simulink model "untitled"  (R2020a)
settings: Solver=VariableStepAuto  StartTime=0.0  StopTime=10.0  RelTol=1e-3
values from neighbouring files (symbols this model uses):
  tmax = 32    [matlab.mat]
  tmin = -26    [matlab.mat]
libraries: mpclib x1
settings Model: Creator=lamarre  LastModifiedBy=lamarre

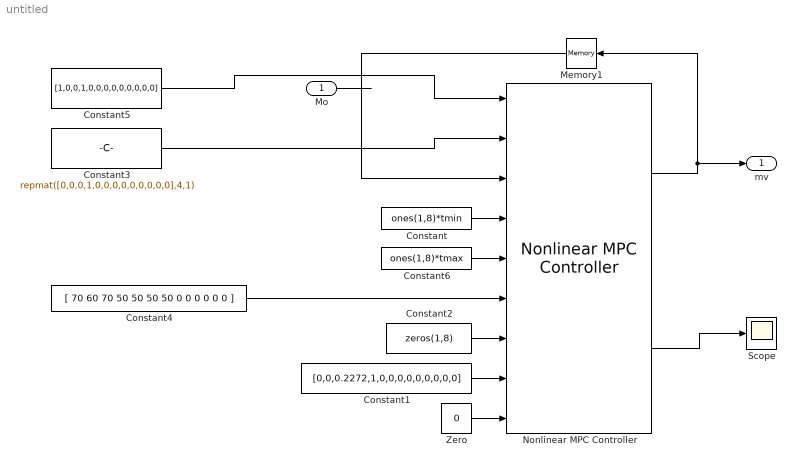
== system untitled ==
  Mo : Inport
  Constant : Constant  Value=ones(1,8)*tmin  VectorParams1D=off
  Constant1 : Constant  Value=[0,0,0.2272,1,0,0,0,0,0,0,0,0,0]  VectorParams1D=off
  Constant2 : Constant  Value=zeros(1,8)  VectorParams1D=off
  Constant3 : Constant  Value=repmat([0,0,0,1,0,0,0,0,0,0,0,0,0],4,1)  VectorParams1D=off
  Constant4 : Constant  Value=[ 70 60 70 50 50 50 50 0 0 0 0 0 0 ]  VectorParams1D=off
  Constant5 : Constant  Value=[1,0,0,1,0,0,0,0,0,0,0,0,0]
  Constant6 : Constant  Value=ones(1,8)*tmax  VectorParams1D=off
  Memory1 : Memory  InitialCondition=[0,0,0,0,0,0,0,0].'
  Nonlinear MPC Controller : mpclib/Nonlinear MPC Controller  SCDEnableBlockLinearizationSpecification=on  nlmpcobj=nlobj  UseObjectTs=on  UseMEX=on  mexname='AUVController'  md_enabled=off  mvtarget_enabled=off  param_enabled=off  cost_enabled=off  mvseq_enabled=off  stateseq_enabled=off  ovseq_enabled=off  slack_enabled=off  status_enabled=on  ov_min=off  ov_max=off  mv_min=on  mv_max=on  mvrate_min=off  mvrate_max=off  state_min=off  state_max=off  ov_weight=on  mv_weight=off  mvrate_weight=off  ecr_weight=off  nlp_initialize=on
  Scope : Scope
  Zero : Constant  Value=0  OutDataTypeStr=Inherit: Inherit via back propagation
  mv : Outport
  wires:
  Constant/1 -> Nonlinear MPC Controller/4
  Nonlinear MPC Controller/2 -> Scope/1
  Constant1/1 -> Nonlinear MPC Controller/8
  Constant2/1 -> Nonlinear MPC Controller/7
  Constant6/1 -> Nonlinear MPC Controller/5
  Zero/1 -> Nonlinear MPC Controller/9
  Constant3/1 -> Nonlinear MPC Controller/2
  Memory1/1 -> Nonlinear MPC Controller/3
  Constant4/1 -> Nonlinear MPC Controller/6
  Nonlinear MPC Controller/1 -> mv/1, Memory1/1
  Mo/1 -> ?
  Constant5/1 -> Nonlinear MPC Controller/1
